simulink library "csbenchlab_dist"  (R2024a)
settings: Solver=VariableStepAuto  StartTime=0.0  StopTime=10.0  RelTol=1e-3
undefined symbols (not defined in the file or in its folder): ZeroNoise_data, ZeroNoise_DT, ZeroNoise_params, ZeroNoise_PT
settings Model: Creator=luka  LastModifiedBy=luka

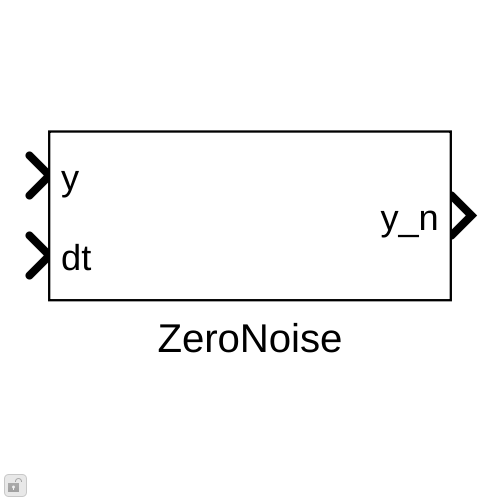
[thumbnail: Simulink's stored preview of the top-level diagram]
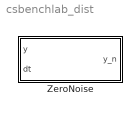
== system csbenchlab_dist ==
  ZeroNoise : Subsystem  Tag=__cs_m_dist;  mask{params=ZeroNoise_params, data=ZeroNoise_data, ParamsType=ZeroNoise_PT, DataType=ZeroNoise_DT}
      mask prompts: params "Parameter struct:"

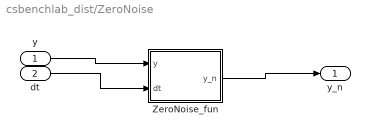
== system csbenchlab_dist/ZeroNoise ==
  y : Inport
  dt : Inport  Port=2
  ZeroNoise_fun : MATLAB Function  TreatAsAtomicUnit=on
  y_n : Outport
  wires:
  y/1 -> ZeroNoise_fun/1(y)
  dt/1 -> ZeroNoise_fun/2(dt)
  ZeroNoise_fun/1(y_n) -> y_n/1

== matlab function csbenchlab_dist/ZeroNoise/ZeroNoise_fun ==
  settings: updateMethod=DISCRETE
  data: y input; y_n output; dt input; data parameter DataType; params parameter ParamsType
% __classname:=ZeroNoise;
function y_n = fcn(y, dt, data, params)
  persistent obj
  if isempty(obj)
    obj = ZeroNoise(params, 'Data', data);
    obj = obj.configure();
  end
 [obj, y_n] = obj.step(y, dt);
end
